simulink model "mconversionFixPointSupport"  (Simulink 6.0)
settings: Solver=FixedStepDiscrete  SolverMode=SingleTasking  StartTime=0.0  StopTime=0.9985  FixedStep=0.001  RelTol=1e-3  AbsTol=1e-6
libraries: simulink x1
settings Model: RequirementInfo=9  CovMetricSettings=d  MinMaxOverflowLogging=MinMaxAndOverflow  Creator=andyb  LastModifiedBy=awarlock  AccelMakeCommand=make_rtw WARN_ON_GLNX=1  ExtModeTrigMode=oneshot  ExtModeArmWhenConnect=off  ExtModeAutoUpdateStatusClock=off
settings DataIOCC: LimitDataPoints=off  OutputSaveName=yout1,yout2,yout3,yout4  SignalLoggingName=sigsOut
settings OptimizationCC: BooleanDataType=off  InlineParams=on
settings DebuggingCC: CheckExecutionContextPreStartOutputMsg=on  CheckExecutionContextRuntimeOutputMsg=on  SolverPrmCheckMsg=none  IntegerOverflowMsg=none  ParameterDowncastMsg=warning  ParameterOverflowMsg=warning  ParameterPrecisionLossMsg=none
settings HardwareCC: TargetUnknown=on
settings RTWCC: TLCAssert=on

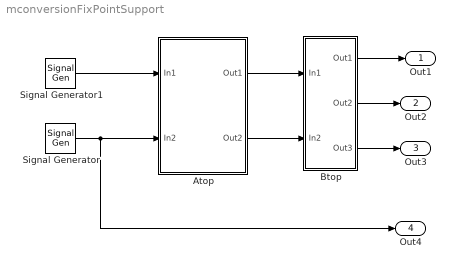
== system mconversionFixPointSupport ==
  Atop : Subsystem  TreatAsAtomicUnit=on  PropExecContextAcrossSSBoundary=on
  Btop : Subsystem  TreatAsAtomicUnit=on  PropExecContextAcrossSSBoundary=on
  Signal Generator : SignalGenerator  WaveForm=sawtooth  Amplitude=5
  Signal Generator1 : SignalGenerator  Frequency=10
  Out1 : Outport
  Out2 : Outport  Port=2
  Out3 : Outport  Port=3
  Out4 : Outport  Port=4
  wires:
  Signal Generator1/1 -> Atop/1(In1)
  Signal Generator/1 -> Out4/1, Atop/2(In2)
  Btop/2(Out2) -> Out2/1
  Btop/1(Out1) -> Out1/1
  Btop/3(Out3) -> Out3/1
  Atop/1(Out1) -> Btop/1(In1)
  Atop/2(Out2) -> Btop/2(In2)

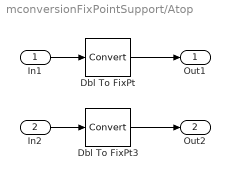
== system mconversionFixPointSupport/Atop ==
  In1 : Inport  Port=1  LatchInput=off
  In2 : Inport  Port=2  LatchInput=off
  Dbl To FixPt : DataTypeConversion  OutDataTypeMode=Specify via dialog  OutDataType=ufix( 8)  OutScaling=2^(-9)  RndMeth=Nearest  SaturateOnIntegerOverflow=on
  Dbl To FixPt3 : DataTypeConversion  OutDataTypeMode=Specify via dialog  OutDataType=sfix(8)  OutScaling=2^(-9)  SaturateOnIntegerOverflow=on
  Out1 : Outport
  Out2 : Outport  Port=2
  wires:
  In2/1 -> Dbl To FixPt3/1
  In1/1 -> Dbl To FixPt/1
  Dbl To FixPt/1 -> Out1/1
  Dbl To FixPt3/1 -> Out2/1

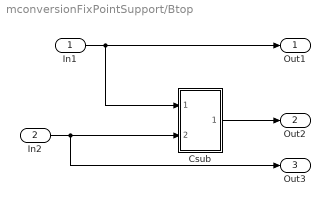
== system mconversionFixPointSupport/Btop ==
  In1 : Inport  Port=1  LatchInput=off
  In2 : Inport  Port=2  LatchInput=off
  Csub : Subsystem  TreatAsAtomicUnit=on  PropExecContextAcrossSSBoundary=on
  Out1 : Outport
  Out2 : Outport  Port=2
  Out3 : Outport  Port=3
  wires:
  In1/1 -> Csub/1(In1), Out1/1
  In2/1 -> Csub/2(In2), Out3/1
  Csub/1(Out1) -> Out2/1

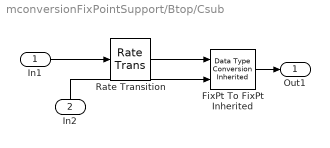
== system mconversionFixPointSupport/Btop/Csub ==
  In1 : Inport  Port=1  LatchInput=off
  In2 : Inport  Orientation=up  Port=2  LatchInput=off
  FixPt To FixPt Inherited : simulink/Signal Attributes/Data Type Conversion Inherited  ConvertRealWorld=Real World Value  RndMeth=Nearest  DoSatur=on
  Rate Transition : RateTransition
  Out1 : Outport
  wires:
  In1/1 -> Rate Transition/1
  In2/1 -> FixPt To FixPt Inherited/2
  FixPt To FixPt Inherited/1 -> Out1/1
  Rate Transition/1 -> FixPt To FixPt Inherited/1
